simulink model "teleoperation_send_pressure_back"  (R2021a)
settings: Solver=VariableStepAuto  StartTime=0.0  StopTime=inf  RelTol=1e-3
model workspace (MATLAB code in the model file):
  | %config file for Matlab server for Matlab-unity communication
  | %%%THIS PART IS INPUT THAT IS OK TO CHANGE TO YOUR NEEDS%%%
  | IPAddress = '127.0.0.1';                            %address for Matlab-Unity communication. 127.0.0.1 means local
  | PiAddress = '131.155.230.140';
  | portNr = 26950;                                     %make sure that this port matches the one chosen in Unity
  | portPi = 12346;
  | nrMessages = 1;                                     %nr of values that you are reading in per packet. Depends on your Unity settings
  | sampleFrequency = 120;                              %frequency on Simulink checking TCP connection
  | 
  | %%%THIS PART YOU ONLY HAVE TO TOUCH WHEN THE UNITY MESSAGE TYPE OR HEADER CHANGES%%
  | headerWidth = 12;                                   %nr of bytes in message header (before actual message)
  | signalWidth = 8;                                    %length of each value in message, depends on data type (which is double for now, which is 8 bytes)
  | messageWidth = nrMessages .* signalWidth;           %length of message without header
  | totalMessageWidth = headerWidth + messageWidth;     %length of total packet
  | sampleTime = 1/sampleFrequency;
values from neighbouring files (symbols this model uses):
  f = [1:0.02:7.02]    [Modulating_sine.m]
libraries: slrealtimeutilitieslib x4, etargetslib x4, slrealtimeiplib x3, instrumentlib x2
settings Model: EnablePacing=on  Creator=slacker  LastModifiedBy=20210123
settings SolverCC: AlgebraicLoopSolver=TrustRegion
settings DebuggingCC: SFMachineParentedDataDiag=warning

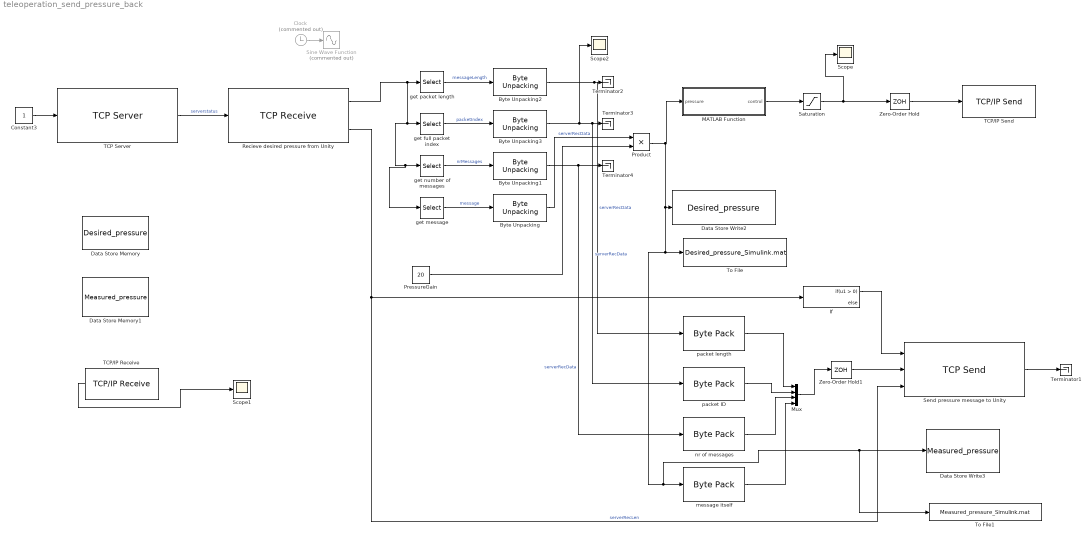
== system teleoperation_send_pressure_back ==
  Byte Unpacking{,1..3} (4 alike) : slrealtimeutilitieslib/Byte Unpacking
      settings: SourceProductBaseCode=XP
  Clock : Clock  Commented=on
  Constant3 : Constant  OutDataTypeStr=double
  Data Store Memory : DataStoreMemory  DataStoreName=Desired_pressure  ReadBeforeWriteMsg=warning  WriteAfterWriteMsg=warning  WriteAfterReadMsg=warning  ShowAdditionalParam=off
  Data Store Memory1 : DataStoreMemory  DataStoreName=Measured_pressure  ReadBeforeWriteMsg=warning  WriteAfterWriteMsg=warning  WriteAfterReadMsg=warning  ShowAdditionalParam=off
  Data Store Write2 : DataStoreWrite  DataStoreName=Desired_pressure  IndexOptions=Index vector (dialog)  Indices=1  OutputSizes=1
  Data Store Write3 : DataStoreWrite  DataStoreName=Measured_pressure  IndexOptions=Index vector (dialog)  Indices=1  OutputSizes=1
  If : If
  MATLAB Function : MATLAB Function  TreatAsAtomicUnit=on
  Mux : Mux
  PressureGain : Constant  Value=20
  Product : Product
  Recieve desired pressure from Unity : slrealtimeiplib/TCP Receive  Priority=1  socketAddPortVal=Server: IPAddress:portNr  rcvWidth=totalMessageWidth  sampleTime=sampleTime
      settings: SourceProductBaseCode=XP
  Saturation : Saturate  UpperLimit=0.7  LowerLimit=0
  Scope : Scope
  Scope1 : Scope
  Scope2 : Scope
  Send pressure message to Unity : slrealtimeiplib/TCP Send  socketAddPortVal=Server: IPAddress:portNr  sampleTime=-1
      settings: SourceProductBaseCode=XP
  Sine Wave Function : Sin  Commented=on  TimeSource=Use external signal  Amplitude=.2  Bias=0.6  Frequency=2  SampleTime=0
  TCP Server : slrealtimeiplib/TCP Server  Priority=-1  useHostTargetConn=off  serverAddress=IPAddress  serverPort=portNr
      settings: SourceProductBaseCode=XP
  TCP/IP Receive : instrumentlib/TCP//IP Receive  Priority=2  Host=131.155.230.140  Port=portPi  DataSize=1  EnableBlockingMode=on  Timeout=0.5  SampleTime=sampleTime  DataType=double  ByteOrder=LittleEndian  ASCIIFormatting=%f,  Terminator=LF
  TCP/IP Send : instrumentlib/TCP//IP Send  Priority=1  Host=131.155.230.140  Port=portPi  EnableBlockingMode=on  Timeout=0.5  ByteOrder=LittleEndian  TransferDelay=on
  Terminator{1..4} (4 alike) : Terminator
  To File : ToFile  Filename=Desired_pressure_Simulink.mat  SaveFormat=Timeseries
  To File1 : ToFile  Filename=Measured_pressure_Simulink.mat  SaveFormat=Timeseries
  Zero-Order Hold : ZeroOrderHold  SampleTime=0.004
  Zero-Order Hold1 : ZeroOrderHold  SampleTime=0.004
  get full packet index : Selector  InputPortWidth=totalMessageWidth  IndexOptions=Index vector (dialog)  Indices=[5:8]  OutputSizes=1
  get message : Selector  InputPortWidth=totalMessageWidth  IndexOptions=Index vector (dialog)  Indices=[headerWidth+1:totalMessageWidth]  OutputSizes=1
  get number of messages : Selector  InputPortWidth=totalMessageWidth  IndexOptions=Index vector (dialog)  Indices=[9:headerWidth]  OutputSizes=1
  get packet length : Selector  InputPortWidth=totalMessageWidth  IndexOptions=Index vector (dialog)  Indices=[1:4]  OutputSizes=1
  message itself : etargetslib/Byte Pack  datatypes={'double'}  byteAlign=1
  nr of messages : etargetslib/Byte Pack  datatypes={'int32'}  byteAlign=1
  packet ID : etargetslib/Byte Pack  datatypes={'int32'}  byteAlign=1
  packet length : etargetslib/Byte Pack  datatypes={'int32'}  byteAlign=1
  wires:
  Saturation/1 -> Zero-Order Hold/1, Scope/1
  Zero-Order Hold/1 -> TCP/IP Send/1
  get number of messages/1 -> Byte Unpacking1/1  "nrMessages"
  get full packet index/1 -> Byte Unpacking3/1  "packetIndex"
  Recieve desired pressure from Unity/2 -> Send pressure message to Unity/3, If/1  "serverRecLen"
  Byte Unpacking2/1 -> packet length/1, Terminator2/1  "serverRecData"
  get packet length/1 -> Byte Unpacking2/1  "messageLength"
  Byte Unpacking3/1 -> Scope2/1, packet ID/1, Terminator3/1  "serverRecData"
  Byte Unpacking1/1 -> nr of messages/1, Terminator4/1  "serverRecData"
  TCP Server/1 -> Recieve desired pressure from Unity/1  "serverstatus"
  get message/1 -> Byte Unpacking/1  "message"
  Constant3/1 -> TCP Server/1
  packet length/1 -> Mux/1
  packet ID/1 -> Mux/2
  Mux/1 -> Zero-Order Hold1/1
  Send pressure message to Unity/1 -> Terminator1/1
  message itself/1 -> Mux/4
  nr of messages/1 -> Mux/3
  PressureGain/1 -> Product/2
  Product/1 -> To File1/1, Data Store Write3/1, message itself/1, To File/1, Data Store Write2/1, MATLAB Function/1(pressure)
  MATLAB Function/1(control) -> Saturation/1
  Recieve desired pressure from Unity/1 -> get message/1, get number of messages/1, get full packet index/1, get packet length/1
  TCP/IP Receive/1 -> Scope1/1
  Clock/1 -> Sine Wave Function/1
  Zero-Order Hold1/1 -> Send pressure message to Unity/2
  Byte Unpacking/1 -> Product/1  "serverRecData"
  If/1 -> Send pressure message to Unity/1

== matlab function teleoperation_send_pressure_back/MATLAB Function ==
  data: pressure input; control output
function control = pressureToPiSignal(pressure)

kPa_min = -100;
kPa_max = 100;
kPa_atmosphere = 100;

control = (kPa_atmosphere + pressure)/(kPa_max - kPa_min);

end
